simulink model "on_line_ciagly"  (R2019b)
settings: Solver=VariableStepAuto  StartTime=0.0  StopTime=20  RelTol=1e-3
libraries: ctrlSharedLib x1
settings Model: Creator=Dominik  LastModifiedBy=a.kuligowski
settings DataIOCC: ReturnWorkspaceOutputs=off
settings DebuggingCC: ArithmeticOperatorsInVariantConditions=warning
settings SFSimCC: SimUseLocalCustomCode=off  CustomCodeUndefinedFunction=UseInterfaceOnly
settings RTWCC: RTWUseLocalCustomCode=off

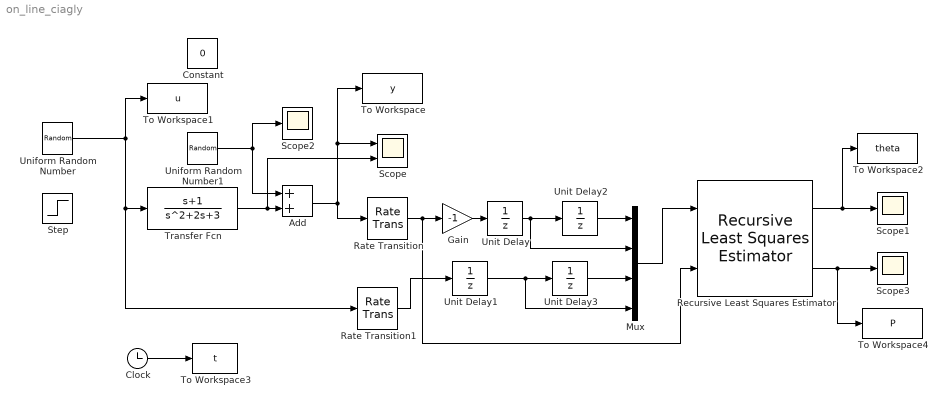
== system on_line_ciagly ==
  Add : Sum
  Clock : Clock
  Constant : Constant  Value=0
  Gain : Gain  Gain=-1
  Mux : Mux
  Rate Transition : RateTransition
  Rate Transition1 : RateTransition
  Recursive Least Squares Estimator : ctrlSharedLib/Recursive Least Squares Estimator  InitialEstimateSource=None  InitialParameterData=4  P0=1000000000  InitialRegressors=0  InitialOutputs=0  History=Infinite  WindowLength=200  EstimationMethod=Forgetting Factor  AdaptationParameter=1  HasTimeVaryingAdaptationParameter=off  NormalizationBias=eps  OutputError=off  OutputP=on  AddEnablePort=off  InputProcessing=Sample-based  Ts=-1
      settings: SourceProductName=Control System Toolbox  SourceProductBaseCode=CT
  Scope : Scope  NumInputPorts=2
  Scope1 : Scope
  Scope2 : Scope
  Scope3 : Scope
  Step : Step  SampleTime=0
  To Workspace : ToWorkspace  VariableName=y  SampleTime=-1
  To Workspace1 : ToWorkspace  VariableName=u  SampleTime=-1
  To Workspace2 : ToWorkspace  VariableName=theta  SampleTime=-1
  To Workspace3 : ToWorkspace  VariableName=t  SampleTime=-1
  To Workspace4 : ToWorkspace  VariableName=P  SampleTime=-1
  Transfer Fcn : TransferFcn  Numerator=[1 1]  Denominator=[1 2 3]
  Uniform Random Number : UniformRandomNumber  SampleTime=0.1
  Uniform Random Number1 : UniformRandomNumber  Minimum=-0.005  Maximum=0.005  Seed=426  SampleTime=0.1
  Unit Delay{,1..3} (4 alike) : UnitDelay  SampleTime=-1  HasFrameUpgradeWarning=on
  wires:
  Transfer Fcn/1 -> Scope/2, Add/2
  Gain/1 -> Unit Delay/1
  Unit Delay/1 -> Mux/2, Unit Delay2/1
  Unit Delay1/1 -> Mux/4, Unit Delay3/1
  Uniform Random Number/1 -> Rate Transition1/1, Transfer Fcn/1, To Workspace1/1
  Mux/1 -> Recursive Least Squares Estimator/1
  Recursive Least Squares Estimator/1 -> To Workspace2/1, Scope1/1
  Clock/1 -> To Workspace3/1
  Recursive Least Squares Estimator/2 -> Scope3/1, To Workspace4/1
  Unit Delay2/1 -> Mux/1
  Unit Delay3/1 -> Mux/3
  Uniform Random Number1/1 -> Scope2/1, Add/1
  Add/1 -> Rate Transition/1, To Workspace/1, Scope/1
  Rate Transition/1 -> Recursive Least Squares Estimator/2, Gain/1
  Rate Transition1/1 -> Unit Delay1/1
